simulink model "gmsk_rx"  (Simulink 7.9)
settings: Solver=FixedStepDiscrete  SolverMode=SingleTasking  StartTime=0.0  StopTime=10.0  RelTol=1e-3
undefined symbols (not defined in the file or in its folder): N
libraries: shlslibv1 x11
settings Model: synDspstartup=OK  Creator=sszilvasi  LastModifiedBy=sszilvasi
settings DataIOCC: SaveOutput=off  SignalLogging=off  SaveTime=off
settings OptimizationCC: InlineParams=on
settings DebuggingCC: AlgebraicLoopMsg=error

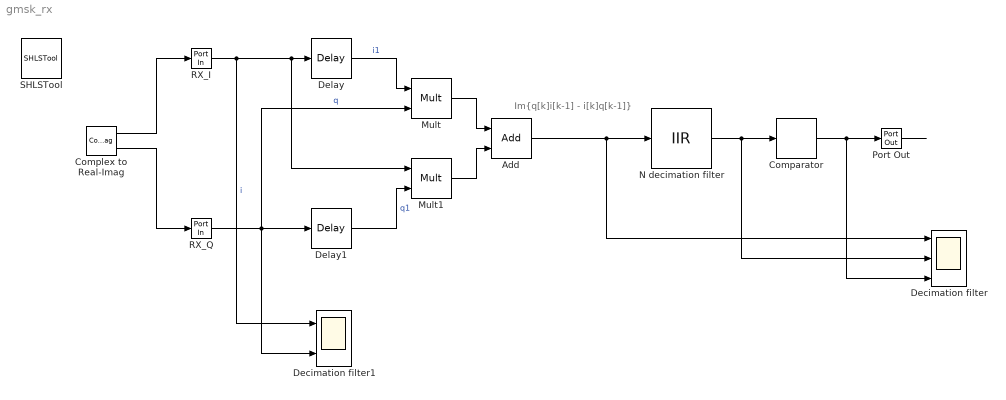
== system gmsk_rx ==
  note: Im{q[k]i[k-1] - i[k]q[k-1]}
  Add : shlslibv1/Math Functions/Add  syn_add_opr=+-  syn_out_f=Full Precision  syn_out_wl=2  syn_out_fl=0  syn_out_dt=signed  syn_out_sat=off  syn_out_rnd=Floor (Truncate)  synBlockType=primitive  synLatency=0  synBlockId=96  syn_sum_of_rows=off
  Comparator : shlslibv1/Math Functions/Comparator  syn_comp_opr=a>=b  syn_comp_const=on  syn_comp_val=0  synBlockType=primitive  synLatency=0  synBlockId=14
  Complex to Real-Imag : ComplexToRealImag  SampleTime=1/8
  Decimation filter : Scope  NumInputPorts=3
      settings: YMin=-5~-5~-5  YMax=5~5~5
  Decimation filter1 : Scope  NumInputPorts=2
      settings: YMin=-5~-5  YMax=5~5
  Delay : shlslibv1/Memories/Delay  syn_delay_val=1  synBlockType=primitive  synLatency=1  synBlockId=104
  Delay1 : shlslibv1/Memories/Delay  syn_delay_val=1  synBlockType=primitive  synLatency=1  synBlockId=104
  Mult : shlslibv1/Math Functions/Mult  syn_out_f=Full Precision  syn_out_wl=16  syn_out_fl=8  syn_out_dt=signed  syn_out_sat=off  syn_out_rnd=Floor (Truncate)  synBlockType=primitive  synLatency=0  synBlockId=3  syn_opr_mode=1
  Mult1 : shlslibv1/Math Functions/Mult  syn_out_f=Full Precision  syn_out_wl=16  syn_out_fl=8  syn_out_dt=signed  syn_out_sat=off  syn_out_rnd=Floor (Truncate)  synBlockType=primitive  synLatency=0  synBlockId=3  syn_opr_mode=1
  N decimation filter : shlslibv1/Filtering/IIR  syn_coefb_vec=[1 zeros(1,N-2) -1]/N  syn_coefa_vec=[1 -1]  syn_coef_fl=8  syn_coef_rnd=on  syn_show_q=off  syn_out_f=Automatic  syn_out_wl=16  syn_out_fl=8  syn_out_dt=signed  syn_out_sat=off  syn_out_rnd=Floor (Truncate)  synBlockType=primitive  synLatency=0  synBlockId=83
  Port Out : shlslibv1/Ports & Subsystems/Port Out  syn_capture=off  syn_register=on  synBlockType=port  synLatency=1  synBlockId=1
  RX_I : shlslibv1/Ports & Subsystems/Port In  syn_out_wl=10  syn_out_fl=9  syn_out_dt=signed  syn_out_st=-1  syn_capture=off  syn_register=off  syn_out_sat=off  syn_out_rnd=off  synBlockType=port  synLatency=0  synBlockId=0
  RX_Q : shlslibv1/Ports & Subsystems/Port In  syn_out_wl=10  syn_out_fl=9  syn_out_dt=signed  syn_out_st=-1  syn_capture=off  syn_register=off  syn_out_sat=off  syn_out_rnd=off  synBlockType=port  synLatency=0  synBlockId=0
  SHLSTool : shlslibv1/SHLSTool  synBlockType=tool  syn_dsp_mode=FPGA
  wires:
  Complex to Real-Imag/1 -> RX_I/1
  Complex to Real-Imag/2 -> RX_Q/1
  RX_Q/1 -> Mult/2, Delay1/1, Decimation filter1/2  "q"
  RX_I/1 -> Delay/1, Mult1/1, Decimation filter1/1  "i"
  Delay/1 -> Mult/1  "i1"
  Delay1/1 -> Mult1/2  "q1"
  Mult/1 -> Add/1
  Mult1/1 -> Add/2
  Add/1 -> N decimation filter/1, Decimation filter/1
  ? -> Complex to Real-Imag/1
  N decimation filter/1 -> Decimation filter/2, Comparator/1
  Comparator/1 -> Decimation filter/3, Port Out/1
  Port Out/1 -> ?
